simulink model "s1"  (Simulink 2.00)
settings: Solver=ode45  StartTime=0.0  StopTime=0.05  MaxStep=0.01  RelTol=1e-5  AbsTol=1e-6
settings Model: SaveTime=off  SaveOutput=off  ConsistencyChecking=off

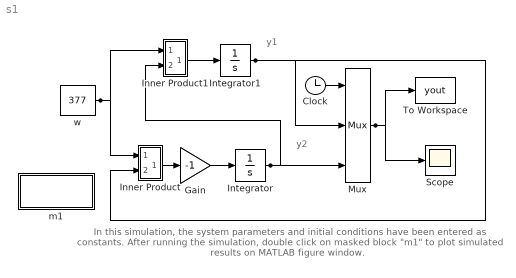
== system s1 ==
  note: In this simulation, the  system parameters and initial conditions have been
      | entered as constants.  After running the simulation, double click on masked
      | block "m1" to plot simulated  results on MATLAB figure window.
  note: y2
  note: y1
  Clock : Clock
      settings: DeleteFcn=simclock BlockIsBeingDestroyed  PostSaveFcn=simclock Save
  m1 : Subsystem
      settings: OpenFcn=m1
      mask Type: Masked block of m1.m
      mask Help: Uses m1.m
      mask Display: disp('Plot yout ')
  Gain : Gain  Gain=-1
  Inner Product : Subsystem
      mask Type: Dot Product
      mask Description:
      | Inner (dot) product.
      | y=sum(u1.*u2)
      mask Help: Computes the inner (dot) product of the inputs: sum(u1.*u2).  The inputs are vectors of the same length. Output is a scalar.
      mask Display: disp('.\n')
  Inner Product1 : Subsystem
      mask Type: Dot Product
      mask Description:
      | Inner (dot) product.
      | y=sum(u1.*u2)
      mask Help: Computes the inner (dot) product of the inputs: sum(u1.*u2).  The inputs are vectors of the same length. Output is a scalar.
      mask Display: disp('.\n')
  Integrator : Integrator  ExternalReset=none  InitialConditionSource=internal  InitialCondition=0  LimitOutput=off  UpperSaturationLimit=inf  LowerSaturationLimit=-inf  ShowSaturationPort=off  ShowStatePort=off  AbsoluteTolerance=auto
  Integrator1 : Integrator  ExternalReset=none  InitialConditionSource=internal  InitialCondition=5  LimitOutput=off  UpperSaturationLimit=inf  LowerSaturationLimit=-inf  ShowSaturationPort=off  ShowStatePort=off  AbsoluteTolerance=auto
  Mux : Mux  Inputs=3
  Scope : Scope
      settings: TickLabels=on  TimeRange=0.05  YMin=-5  YMax=5  SaveToWorkspace=off  SaveName=ScopeData
  To Workspace : ToWorkspace  VariableName=yout  SampleTime=0
      settings: Buffer=3000
  w : Constant  Value=377
  wires:
  w/1 -> Inner Product/1(in_1), Inner Product1/1(in_1)
  Inner Product1/1(out_1) -> Integrator1/1
  Mux/1 -> To Workspace/1, Scope/1
  Inner Product/1(out_1) -> Gain/1
  Gain/1 -> Integrator/1
  Clock/1 -> Mux/1
  Integrator1/1 -> Inner Product/2(in_2), Mux/2
  Integrator/1 -> Inner Product1/2(in_2), Mux/3

== system s1/m1 ==
  note: Uses m1.m to plot the simulated result
      | stored in yout of  the Matlab workspace

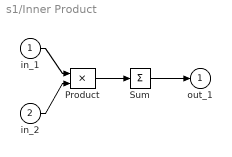
== system s1/Inner Product ==
  in_1 : Inport  Port=1  PortWidth=-1  SampleTime=-1
  in_2 : Inport  Port=2  PortWidth=-1  SampleTime=-1
  Product : Product  Inputs=2
  Sum : Sum  Inputs=+
  out_1 : Outport  Port=1  InitialOutput=0
  wires:
  in_2/1 -> Product/2
  in_1/1 -> Product/1
  Product/1 -> Sum/1
  Sum/1 -> out_1/1

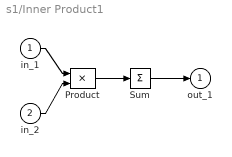
== system s1/Inner Product1 ==
  in_1 : Inport  Port=1  PortWidth=-1  SampleTime=-1
  in_2 : Inport  Port=2  PortWidth=-1  SampleTime=-1
  Product : Product  Inputs=2
  Sum : Sum  Inputs=+
  out_1 : Outport  Port=1  InitialOutput=0
  wires:
  in_2/1 -> Product/2
  in_1/1 -> Product/1
  Product/1 -> Sum/1
  Sum/1 -> out_1/1
